simulink model "StateSpaceController"  (R2021a)
settings: Solver=VariableStepAuto  StartTime=0.0  StopTime=15  RelTol=1e-3
values from neighbouring files (symbols this model uses):
  Sim_A = m.EquilibriumStateSpace.A    [assignment_Q1.m]    (also in main.m)
  Sim_B = m.EquilibriumStateSpace.B    [assignment_Q1.m]    (also in main.m)
  Sim_C = m.EquilibriumStateSpace.C    [assignment_Q1.m]    (also in main.m)
  Sim_G = G    [assignment_Q1.m]    (also in main.m)
  Sim_K = K    [assignment_Q1.m]    (also in main.m)
  Sim_Kr = Kr    [assignment_Q1.m]    (also in main.m)
settings Model: Creator=james  LastModifiedBy=james

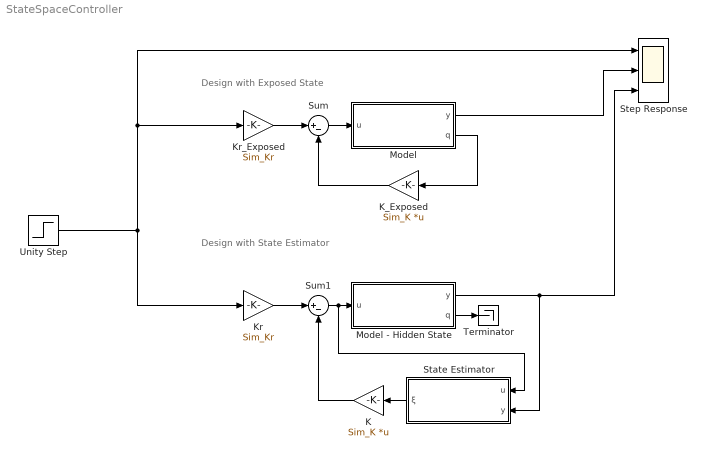
== system StateSpaceController ==
  note: Design with Exposed State
  note: Design with State Estimator
  K : Gain  Gain=Sim_K  Multiplication=Matrix(K*u)
  K_Exposed : Gain  Gain=Sim_K  Multiplication=Matrix(K*u)
  Kr : Gain  Gain=Sim_Kr
  Kr_Exposed : Gain  Gain=Sim_Kr
  Model : Subsystem
  Model - Hidden State : Subsystem
  State Estimator : Subsystem
  Step Response : Scope  NumInputPorts=3
  Sum : Sum  Inputs=|+-
  Sum1 : Sum  Inputs=|+-
  Terminator : Terminator
  Unity Step : Step  SampleTime=0
  wires:
  Sum/1 -> Model/1(u)
  Unity Step/1 -> Step Response/1, Kr_Exposed/1, Kr/1
  K_Exposed/1 -> Sum/2
  Model/2(q) -> K_Exposed/1
  Kr_Exposed/1 -> Sum/1
  Kr/1 -> Sum1/1
  K/1 -> Sum1/2
  Model - Hidden State/1(y) -> Step Response/3, State Estimator/2(y)
  Sum1/1 -> State Estimator/1(u), Model - Hidden State/1(u)
  Model - Hidden State/2(q) -> Terminator/1
  State Estimator/1(ξ) -> K/1
  Model/1(y) -> Step Response/2

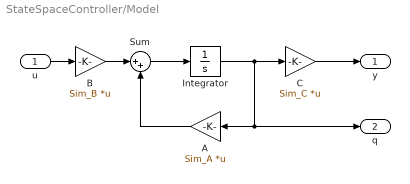
== system StateSpaceController/Model ==
  u : Inport
  A : Gain  Gain=Sim_A  Multiplication=Matrix(K*u)
  B : Gain  Gain=Sim_B  Multiplication=Matrix(K*u)
  C : Gain  Gain=Sim_C  Multiplication=Matrix(K*u)
  Integrator : Integrator
  Sum : Sum  Inputs=|++
  y : Outport
  q : Outport  Port=2
  wires:
  B/1 -> Sum/1
  C/1 -> y/1
  Integrator/1 -> q/1, A/1, C/1
  u/1 -> B/1
  Sum/1 -> Integrator/1
  A/1 -> Sum/2

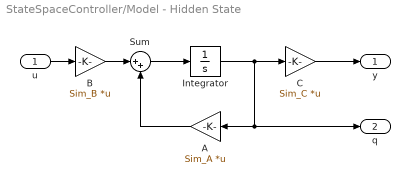
== system StateSpaceController/Model - Hidden State ==
  u : Inport
  A : Gain  Gain=Sim_A  Multiplication=Matrix(K*u)
  B : Gain  Gain=Sim_B  Multiplication=Matrix(K*u)
  C : Gain  Gain=Sim_C  Multiplication=Matrix(K*u)
  Integrator : Integrator
  Sum : Sum  Inputs=|++
  y : Outport
  q : Outport  Port=2
  wires:
  B/1 -> Sum/1
  C/1 -> y/1
  Integrator/1 -> q/1, A/1, C/1
  u/1 -> B/1
  Sum/1 -> Integrator/1
  A/1 -> Sum/2

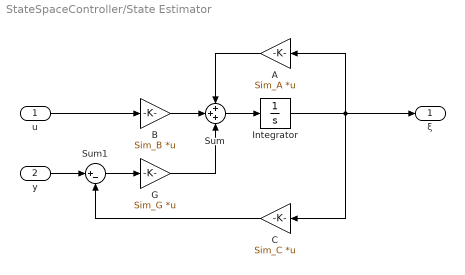
== system StateSpaceController/State Estimator ==
  u : Inport
  y : Inport  Port=2
  A : Gain  Gain=Sim_A  Multiplication=Matrix(K*u)
  B : Gain  Gain=Sim_B  Multiplication=Matrix(K*u)
  C : Gain  Gain=Sim_C  Multiplication=Matrix(K*u)
  G : Gain  Gain=Sim_G  Multiplication=Matrix(K*u)
  Integrator : Integrator
  Sum : Sum  Inputs=+++
  Sum1 : Sum  Inputs=|+-
  ξ : Outport
  wires:
  Integrator/1 -> C/1, A/1, ξ/1
  Sum/1 -> Integrator/1
  B/1 -> Sum/2
  u/1 -> B/1
  C/1 -> Sum1/2
  y/1 -> Sum1/1
  A/1 -> Sum/1
  Sum1/1 -> G/1
  G/1 -> Sum/3
